simulink model "Diff_MOD"  (Simulink 7.9)
settings: Solver=ode45  StartTime=0.0  StopTime=simu.trantime  RelTol=1e-3
undefined symbols (not defined in the file): dc, Fs, mod, OSR, sinamp, sinfreq
libraries: commsynccomp2 x2, dsparch4 x1, simulink x1, dspsrcs4 x1
settings Model: Creator=amyles  LastModifiedBy=Arnaldi Isacco
settings SolverCC: ZcThreshold=1e-3  ZeroCrossAlgorithm=Adaptive  AutoInsertRateTranBlk=on  InsertRTBMode=Always
settings DataIOCC: LimitDataPoints=off  MaxDataPoints=50000  SaveOutput=off  SignalLogging=off  DSMLogging=off  SaveTime=off
settings OptimizationCC: InlineParams=on
settings DebuggingCC: SaveWithDisabledLinksMsg=none  SaveWithParameterizedLinksMsg=none  StrictBusMsg=Warning
settings ModelReferenceCC: ModelReferenceNumInstancesAllowed=Single
settings CodeAppCC: CustomSymbolStrType=$N$R$M_T
settings GRTTargetCC: CombineOutputUpdateFcns=off  GRTInterface=on
settings ConfigurationSet: Description=SimMechanics 2G

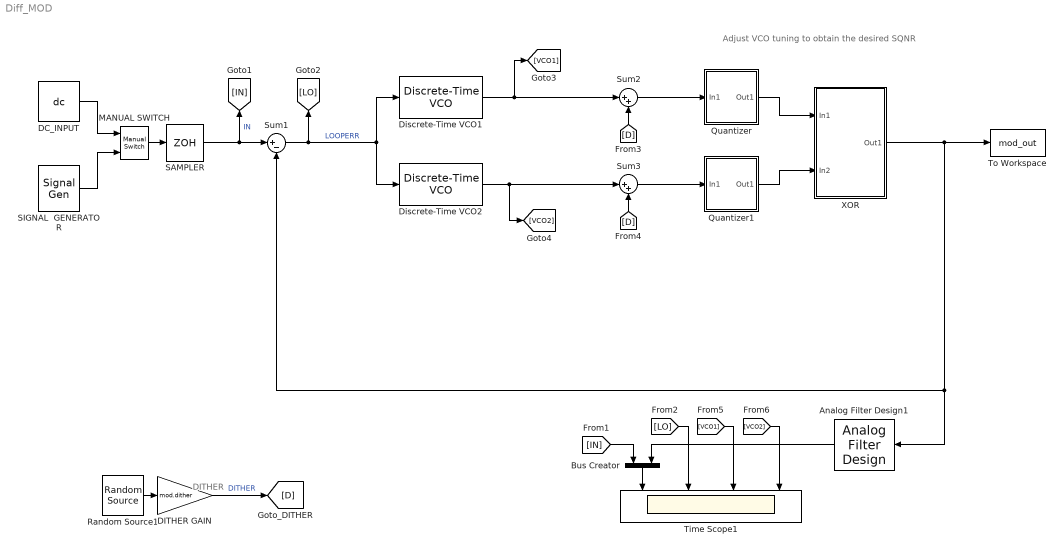
== system Diff_MOD ==
  note: DITHER
  note: Adjust VCO tuning to obtain the desired SQNR
  Analog Filter Design1 : dsparch4/Analog Filter Design  method=Butterworth  filttype=Lowpass  N=8  Wlo=pi*(Fs/OSR)  Whi=80  Rp=2  Rs=40
  Bus Creator : BusCreator  Inputs=2
  DC_INPUT : Constant  Value=dc  OutDataTypeStr=double  SampleTime=1/Fs
  DITHER GAIN : Gain  Gain=mod.dither  SampleTime=1/Fs
  Discrete-Time VCO1 : commsynccomp2/Discrete-Time VCO  Ac=sinamp*2  Fc=Fs/2  Kc=sinfreq*24  Ph=0  ts=1/Fs
  Discrete-Time VCO2 : commsynccomp2/Discrete-Time VCO  Ac=-sinamp*2  Fc=Fs/2  Kc=sinfreq*24  Ph=1.571  ts=1/Fs
  MANUAL SWITCH : simulink/Signal Routing/Manual Switch  sw=0  action=0  varsize=off
      settings: AttributesFormatString=Double click to\nselect the desired\ninput
  Quantizer : Subsystem
  Quantizer1 : Subsystem
  Random Source1 : dspsrcs4/Random Source  SrcType=Uniform  NormMethod=Ziggurat  CltLength=12  MinVal=-1  MaxVal=1  MeanVal=0  VarVal=1  RepMode=Not repeatable  rawSeed=1  IsInherit=off  SampMode=Discrete  SampTime=1/Fs  SampFrame=1  DataType=Double  OutComplex=Real
  SAMPLER : ZeroOrderHold  SampleTime=1/Fs
  SIGNAL  GENERATOR : SignalGenerator  Amplitude=sinamp  Frequency=sinfreq  VectorParams1D=off
  Sum1 : Sum  Inputs=|+-  SampleTime=1/Fs
  Sum2 : Sum  Inputs=|++
  Sum3 : Sum  Inputs=|++
  Time Scope1 : Scope  NumInputPorts=4
      settings: TimeRange=0.01  YMin=-1.1~-3~0~0.15  YMax=1.1~1~2~0.6  DataFormat=Structure  MaxDataPoints=10000
  To Workspace : ToWorkspace  VariableName=mod_out  SampleTime=-1
      settings: AttributesFormatString=Export output to\nworkspace for\npost-processing
  XOR : Subsystem
  wires:
  Sum1/1 -> [LO], Discrete-Time VCO1/1, Discrete-Time VCO2/1  "LOOPERR"
  XOR/1(Out1) -> Analog Filter Design1/1, Sum1/2, To Workspace/1
  Discrete-Time VCO1/1 -> Sum2/1, [VCO1]
  Discrete-Time VCO2/1 -> Sum3/1, [VCO2]
  Quantizer/1(Out1) -> XOR/1(In1)
  Sum2/1 -> Quantizer/1(In1)
  [D] -> Sum2/2
  Quantizer1/1(Out1) -> XOR/2(In2)
  [D] -> Sum3/2
  Sum3/1 -> Quantizer1/1(In1)
  SAMPLER/1 -> Sum1/1, [IN]  "IN"
  Random Source1/1 -> DITHER GAIN/1
  DITHER GAIN/1 -> [D]  "DITHER"
  DC_INPUT/1 -> MANUAL SWITCH/1
  SIGNAL  GENERATOR/1 -> MANUAL SWITCH/2
  MANUAL SWITCH/1 -> SAMPLER/1
  Bus Creator/1 -> Time Scope1/1
  [IN] -> Bus Creator/1
  Analog Filter Design1/1 -> Bus Creator/2
  [LO] -> Time Scope1/2
  [VCO1] -> Time Scope1/3
  [VCO2] -> Time Scope1/4

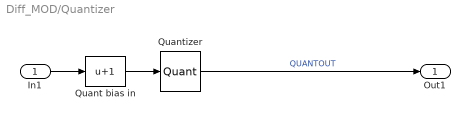
== system Diff_MOD/Quantizer ==
  In1 : Inport
  Quant bias in : Bias  Bias=1
      settings: AttributesFormatString=Need offset to give\nMID-RISE quantiser
  Quantizer : Quantizer  QuantizationInterval=2  SampleTime=1/Fs
      settings: AttributesFormatString=step = 2
  Out1 : Outport
  wires:
  Quant bias in/1 -> Quantizer/1
  Quantizer/1 -> Out1/1  "QUANTOUT"
  In1/1 -> Quant bias in/1

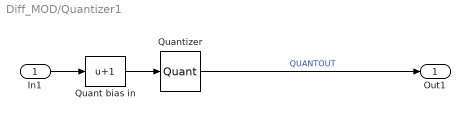
== system Diff_MOD/Quantizer1 ==
  In1 : Inport
  Quant bias in : Bias  Bias=1
      settings: AttributesFormatString=Need offset to give\nMID-RISE quantiser
  Quantizer : Quantizer  QuantizationInterval=2  SampleTime=1/Fs
      settings: AttributesFormatString=step = 2
  Out1 : Outport
  wires:
  Quant bias in/1 -> Quantizer/1
  Quantizer/1 -> Out1/1  "QUANTOUT"
  In1/1 -> Quant bias in/1

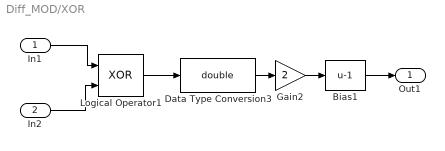
== system Diff_MOD/XOR ==
  In1 : Inport
  In2 : Inport  Port=2
  Bias1 : Bias  Bias=-1
  Data Type Conversion3 : DataTypeConversion  OutDataTypeStr=double  SampleTime=1/Fs
  Gain2 : Gain  Gain=2  SampleTime=1/Fs
  Logical Operator1 : Logic  Operator=XOR  IconShape=distinctive  AllPortsSameDT=off  OutDataTypeStr=boolean  SampleTime=1/Fs
  Out1 : Outport
  wires:
  Logical Operator1/1 -> Data Type Conversion3/1
  Data Type Conversion3/1 -> Gain2/1
  Gain2/1 -> Bias1/1
  Bias1/1 -> Out1/1
  In2/1 -> Logical Operator1/2
  In1/1 -> Logical Operator1/1
